simulink model "q1_hw7"  (R2021b)
settings: Solver=VariableStepAuto  StartTime=0.0  StopTime=50  RelTol=1e-3
settings Model: Creator=Reyhaneh  LastModifiedBy=Reyhaneh

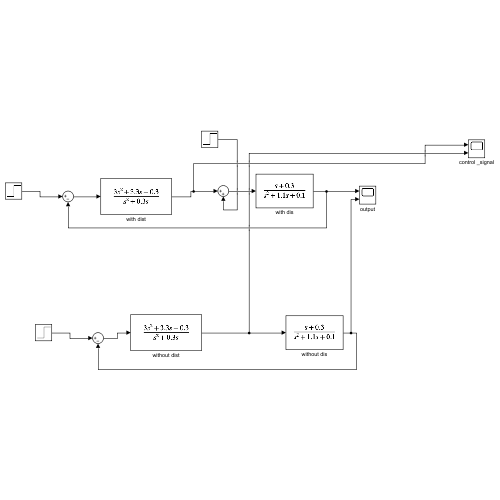
[thumbnail: Simulink's stored preview of the top-level diagram]
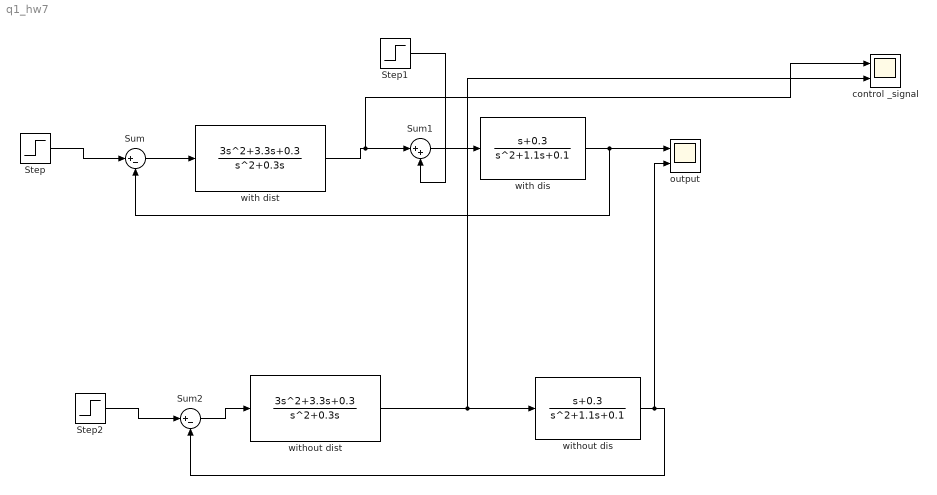
== system q1_hw7 ==
  Step : Step  Time=0  SampleTime=0
  Step1 : Step  Time=0  SampleTime=0
  Step2 : Step  Time=0  SampleTime=0
  Sum : Sum  Inputs=|+-
  Sum1 : Sum  Inputs=|++
  Sum2 : Sum  Inputs=|+-
  control _signal : Scope  NumInputPorts=2
  output : Scope  NumInputPorts=2
  with dis : TransferFcn  Numerator=[1 0.3]  Denominator=[1 1.1 0.1]
  with dist : TransferFcn  Numerator=[3 3.3 0.3]  Denominator=[1 0.3 0]
  without dis : TransferFcn  Numerator=[1 0.3]  Denominator=[1 1.1 0.1]
  without dist : TransferFcn  Numerator=[3 3.3 0.3]  Denominator=[1 0.3 0]
  wires:
  Step/1 -> Sum/1
  Sum/1 -> with dist/1
  with dis/1 -> output/1, Sum/2
  with dist/1 -> control _signal/1, Sum1/1
  Sum1/1 -> with dis/1
  Step1/1 -> Sum1/2
  without dist/1 -> without dis/1, control _signal/2
  Sum2/1 -> without dist/1
  Step2/1 -> Sum2/1
  without dis/1 -> Sum2/2, output/2
